simulink model "main"  (R2022b)
settings: Solver=VariableStepAuto  StartTime=0.0  StopTime=stop_time  FixedStep=Ts  RelTol=1e-3
undefined symbols (not defined in the file): A_c, alpha, B_c, beta, C, D, E, F, H, K, m, n, N, r_z, V, x0
settings Model: Creator=toshi  LastModifiedBy=toshi
settings DebuggingCC: AlgebraicLoopMsg=none

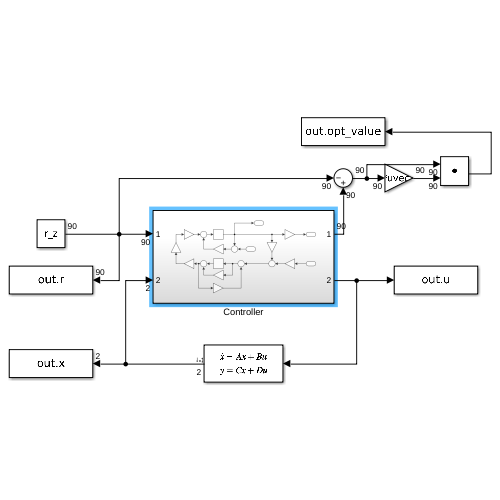
[thumbnail: Simulink's stored preview of the top-level diagram]
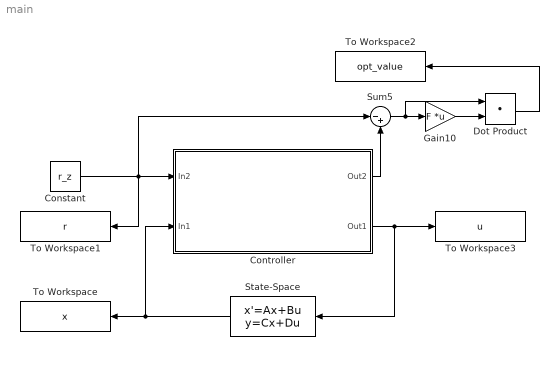
== system main ==
  Constant : Constant  Value=r_z
  Controller : Subsystem
  Dot Product : DotProduct  OutDataTypeStr=Inherit: Inherit via internal rule
  Gain10 : Gain  Gain=F  Multiplication=Matrix(K*u) (u vector)
  State-Space : StateSpace  A=A_c  B=B_c  C=C  D=D  InitialCondition=x0  ParameterTunability=Unconstrained
  Sum5 : Sum  Inputs=|-+
  To Workspace : ToWorkspace  VariableName=x  SaveFormat=Timeseries  SampleTime=-1
  To Workspace1 : ToWorkspace  VariableName=r  SaveFormat=Timeseries  SampleTime=-1
  To Workspace2 : ToWorkspace  VariableName=opt_value  SaveFormat=Timeseries  SampleTime=-1
  To Workspace3 : ToWorkspace  VariableName=u  SaveFormat=Timeseries  SampleTime=-1
  wires:
  State-Space/1 -> To Workspace/1, Controller/2(In1)
  Controller/2(Out1) -> State-Space/1, To Workspace3/1
  Constant/1 -> Sum5/1, To Workspace1/1, Controller/1(In2)
  Controller/1(Out2) -> Sum5/2
  Sum5/1 -> Gain10/1, Dot Product/1
  Gain10/1 -> Dot Product/2
  Dot Product/1 -> To Workspace2/1

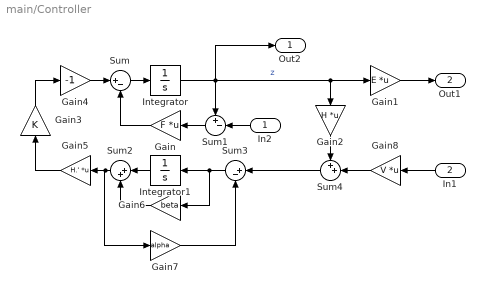
== system main/Controller ==
  In2 : Inport
  In1 : Inport  Port=2
  Gain : Gain  Gain=F  Multiplication=Matrix(K*u) (u vector)
  Gain1 : Gain  Gain=E  Multiplication=Matrix(K*u) (u vector)
  Gain2 : Gain  Gain=H  Multiplication=Matrix(K*u) (u vector)
  Gain3 : Gain  Gain=K
  Gain4 : Gain  Gain=-1
  Gain5 : Gain  Gain=H.'  Multiplication=Matrix(K*u) (u vector)
  Gain6 : Gain  Gain=beta
  Gain7 : Gain  Gain=alpha
  Gain8 : Gain  Gain=V  Multiplication=Matrix(K*u) (u vector)
  Integrator : Integrator  InitialCondition=zeros((m + n) *N, 1)
  Integrator1 : Integrator  InitialCondition=zeros(n * N, 1)
  Sum : Sum  Inputs=|+-
  Sum1 : Sum  Inputs=+-|
  Sum2 : Sum  Inputs=|++
  Sum3 : Sum  Inputs=|+-
  Sum4 : Sum  Inputs=++|
  Out2 : Outport
  Out1 : Outport  Port=2
  wires:
  Integrator/1 -> Gain2/1, Gain1/1, Out2/1, Sum1/1  "z"
  Sum/1 -> Integrator/1
  Gain/1 -> Sum/2
  Gain5/1 -> Gain3/1
  Gain3/1 -> Gain4/1
  Gain4/1 -> Sum/1
  Gain8/1 -> Sum4/2
  Sum1/1 -> Gain/1
  Sum2/1 -> Gain7/1, Gain5/1
  Gain1/1 -> Out1/1
  Gain6/1 -> Sum2/2
  Gain2/1 -> Sum4/1
  Sum4/1 -> Sum3/1
  Integrator1/1 -> Sum2/1
  Sum3/1 -> Gain6/1, Integrator1/1
  Gain7/1 -> Sum3/2
  In2/1 -> Sum1/2
  In1/1 -> Gain8/1
